simulink subsystem "offset_free_MPC"  (R2023a)
settings: Solver=VariableStepAuto  StartTime=0.0  StopTime=10.0  RelTol=1e-3
undefined symbols (not defined in the file): DiscIntNeverNeededParam, offset_free_I_gain
settings Model: Creator=tshintai  LastModifiedBy=tshintai
settings OptimizationCC: ReuseModelBlockBuffer=off
settings ModelReferenceCC: EnableRefExpFcnMdlSchedulingChecks=on

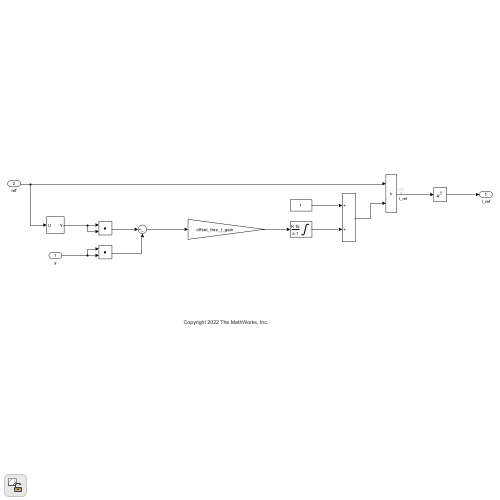
[thumbnail: Simulink's stored preview of the top-level diagram]
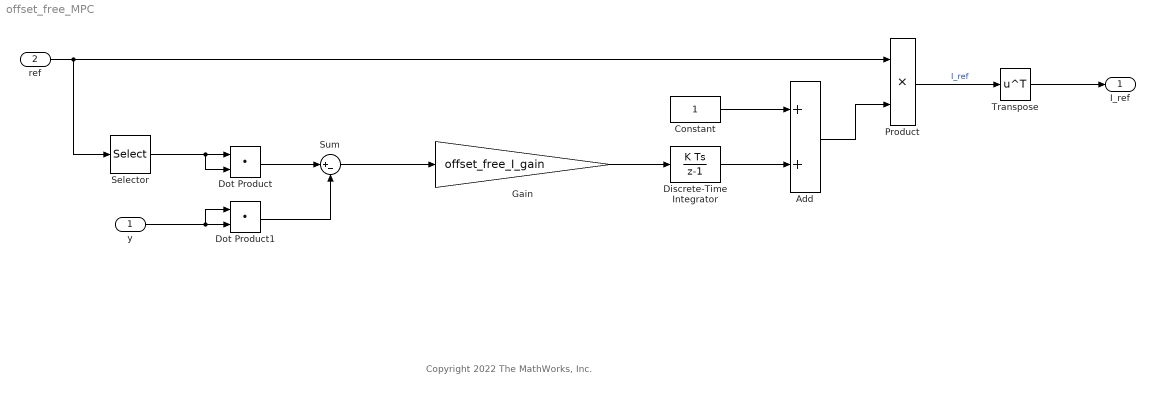
== system offset_free_MPC ==
  note: Copyright 2022 The MathWorks, Inc.
  y : Inport
  ref : Inport  Port=2
  Add : Sum
  Constant : Constant  OutDataTypeStr=single
  Discrete-Time Integrator : DiscreteIntegrator  SampleTime=-1  LimitOutput=on  LowerSaturationLimit=-1  ICPrevOutput=DiscIntNeverNeededParam  ICPrevScaledInput=DiscIntNeverNeededParam
  Dot Product : DotProduct  OutDataTypeStr=Inherit: Inherit via internal rule
  Dot Product1 : DotProduct  OutDataTypeStr=Inherit: Inherit via internal rule
  Gain : Gain  Gain=offset_free_I_gain
  Product : Product
  Selector : Selector  NumberOfDimensions=2  InputPortWidth=3  IndexOptions=Select all,Index vector (dialog)  Indices=[1 3],1  OutputSizes=1,1
  Sum : Sum  Inputs=|+-
  Transpose : Math  Operator=transpose
  I_ref : Outport
  wires:
  ref/1 -> Selector/1, Product/1
  Selector/1 -> Dot Product/1, Dot Product/2
  y/1 -> Dot Product1/1, Dot Product1/2
  Discrete-Time Integrator/1 -> Add/2
  Constant/1 -> Add/1
  Add/1 -> Product/2
  Gain/1 -> Discrete-Time Integrator/1
  Transpose/1 -> I_ref/1
  Product/1 -> Transpose/1  "I_ref"
  Sum/1 -> Gain/1
  Dot Product1/1 -> Sum/2
  Dot Product/1 -> Sum/1
